simulink model "longitudinal_lateral_dynamics"  (R2024b)
settings: Solver=VariableStepAuto  StartTime=0.0  StopTime=10  RelTol=1e-3
values from neighbouring files (symbols this model uses):
  Cd = [0 1]    [mpc3.m]
  Cr = 87342    [mpc3.m]    (also in prueba_mpc.m; prueba_mpc2.m)
  Iz = 1960    [mpc3.m]    (also in prueba_mpc.m; prueba_mpc2.m)
  lf = 1.177    [mpc3.m]    (also in prueba_mpc.m; prueba_mpc2.m)
  lr = 1.358    [mpc3.m]    (also in prueba_mpc.m; prueba_mpc2.m)
  m = 1400    [mpc3.m]    (also in prueba_mpc.m; prueba_mpc2.m)
  R = 1    [prueba_mpc.m]    (also in prueba_mpc2.m)
  vx = 10    [mpc3.m]    (also in prueba_mpc.m; prueba_mpc2.m)
undefined symbols (not defined in the file or in its folder): Af, F_max, FN, g, miu, mode, mu1, mu2, mu3, steering_angle, theta
libraries: slpidlib x1
settings Model: Creator=inaki  LastModifiedBy=inaki
settings SolverCC: MaxConsecutiveMinStep=4
settings DebuggingCC: AlgebraicLoopMsg=none

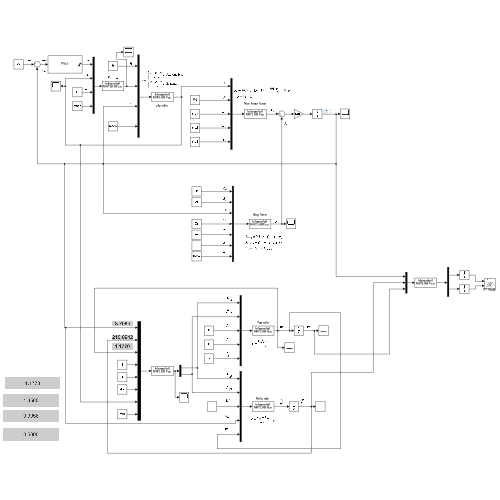
[thumbnail: Simulink's stored preview of the top-level diagram]
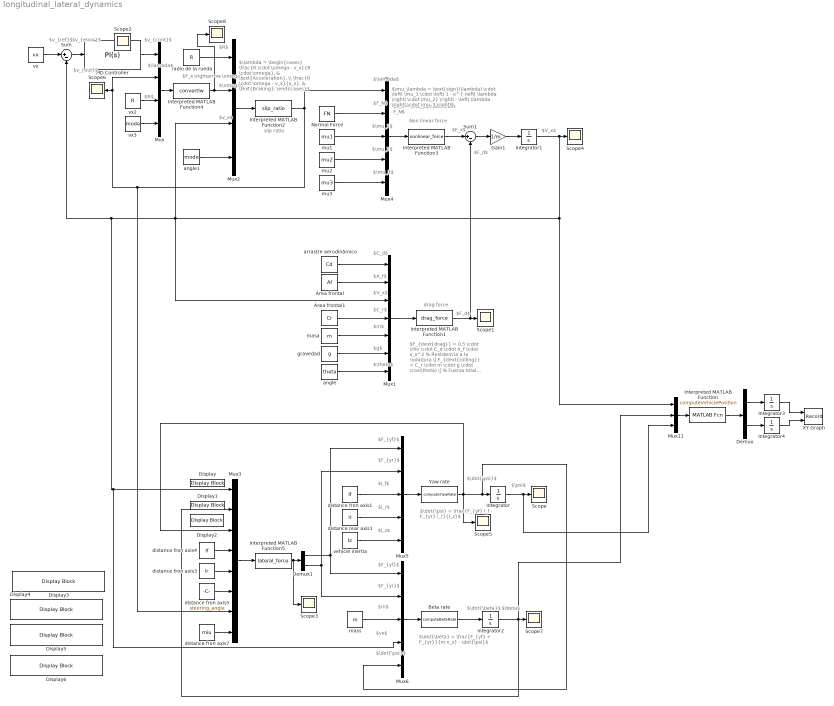
== system longitudinal_lateral_dynamics ==
  note: $v_{out}$
  note: $V_x$
  note: $V_x$
  note: $\mu_1$
  note: slip ratio
  note: $F_x \rightarrow \omega$
  note: $m$
  note: drag force
  note: $v_{error}$
  note: $C_d$
  note: $F_{\text{drag}} = 0.5 \cdot \rho \cdot C_d \cdot A_f \cdot v_x^2 % Resistencia a la rodadura \[ F_{\text{rolling}} = C_r \cdot m \cdot g \cdot \cos(\theta) \] % Fuerza total de arrastre \[ F_D = F_{\text{drag}} + F_{\text{rolling}} \]$
  note: $\lambda$
  note: $F_d$
  note: Non linear force
  note: $\omega$
  note: $F_x = \mu_\lambda \cdot F_N$
  note: $F_d$
  note: $A_f$
  note: $C_r$
  note: $v_{cont}$
  note: $g$
  note: $v_{ref}$
  note: $v_x$
  note: $\theta$
  note: $F_x$
  note: $\lambda = \begin{cases} \frac{R \cdot \omega - v_x}{R \cdot \omega}, & \text{Acceleration}, \\ \frac{R \cdot \omega - v_x}{v_x}, & \text{Braking}. \end{cases}$
  note: $R$
  note: $\lambda$
  note: $\mu_3$
  note: $\mu_\lambda = \text{sign}(\lambda) \cdot \left( \mu_1 \cdot \left( 1 - e^{-\left| \lambda \right| \cdot \mu_2} \right) - \left| \lambda \right| \cdot \mu_3 \right)$
  note: $R$
  note: $\mu_2$
  note: $F_N$
  note: $\dot{\psi}$
  note: $F_{yr}$
  note: $\dot{\beta}$
  note: $F_{yf}$
  note: $\dot{\beta} = \frac{F_{yf} + F_{yr}}{m v_x} - \dot{\psi}$
  note: $m$
  note: $\dot{\psi}$
  note: $F_{yf}$
  note: $vx$
  note: $\psi$
  note: $I_r$
  note: $\beta$
  note: $I_z$
  note: $F_{yr}$
  note: $I_f$
  note: $\dot{\psi} = \frac{F_{yf} l_f - F_{yr} l_r}{I_z}$
  Beta rate : MATLABFcn  MATLABFcn=computeBetaRate
  Demux : Demux  Outputs=2
  Demux1 : Demux  Outputs=2
  Display{,1,3..6} (6 alike) : DisplayBlock  LabelPosition=Hide  Transparency=1
  Display2 : DisplayBlock  LabelPosition=Hide  Transparency=1  Layout=Fill available space
  Gain1 : Gain  Gain=1/m
  Integrator{,1..4} (5 alike) : Integrator
  Interpreted MATLAB Function : MATLABFcn  MATLABFcn=computeVehiclePosition
  Interpreted MATLAB Function1 : MATLABFcn  MATLABFcn=drag_force  Output1D=off
  Interpreted MATLAB Function2 : MATLABFcn  MATLABFcn=slip_ratio  Output1D=off
  Interpreted MATLAB Function3 : MATLABFcn  MATLABFcn=nonlinear_force  Output1D=off
  Interpreted MATLAB Function4 : MATLABFcn  MATLABFcn=convertlw  OutputDimensions=1  Output1D=off
  Interpreted MATLAB Function5 : MATLABFcn  MATLABFcn=lateral_force  OutputDimensions=2
  Mux : Mux
  Mux1 : Mux  Inputs=7
  Mux11 : Mux  Inputs=3
  Mux2 : Mux
  Mux3 : Mux  Inputs=8
  Mux4 : Mux  Inputs=5
  Mux5 : Mux  Inputs=5
  Mux6 : Mux  Inputs=5
  Normal Force : Constant  Value=FN
  PID Controller : slpidlib/PID Controller  Controller=PI  Form=Parallel  TimeDomain=Continuous-time  UseExternalTs=off  SampleTime=-1  IntegratorMethod=Forward Euler  FilterMethod=Forward Euler  ControllerParametersSource=internal  P=3371.8  I=1668.7038  UseKiTs=off  D=0  UseExternalDerivativeSource=off  N=100  UseFilter=on  TunerSelectOption=Transfer Function Based (PID Tuner App)  InitialConditionSource=internal  InitialConditionForIntegrator=0  InitialConditionForFilter=0  DifferentiatorICPrevScaledInput=0  ExternalReset=none  TrackingMode=off  Kt=1  LimitOutput=on  SatLimitsSource=internal  UpperSaturationLimit=F_max  LowerSaturationLimit=-F_max  LinearizeAsGain=on  AntiWindupMode=clamping  Kb=1  LimitIntegrator=off  UpperIntegratorSaturationLimit=inf  LowerIntegratorSaturationLimit=-inf  POutMin=[]  POutMax=[]  IOutMin=[]  IOutMax=[]  DOutMin=[]  DOutMax=[]  NOutMin=[]  NOutMax=[]  SumOutMin=[]  SumOutMax=[]  SaturationOutMin=[]  SaturationOutMax=[]  PParamMin=[]  PParamMax=[]  IParamMin=[]  IParamMax=[]  DParamMin=[]  DParamMax=[]  NParamMin=[]  NParamMax=[]  KbParamMin=[]  KbParamMax=[]  KtParamMin=[]  KtParamMax=[]  KbOutMin=[]  KbOutMax=[]  KtOutMin=[]  KtOutMax=[]  IntegratorOutMin=[]  IntegratorOutMax=[]  FilterOutMin=[]  FilterOutMax=[]  SumI1OutMin=[]  SumI1OutMax=[]  SumI2OutMin=[]  SumI2OutMax=[]  SumI3OutMin=[]  SumI3OutMax=[]  SumI4OutMin=[]  SumI4OutMax=[]  SumDOutMin=[]  SumDOutMax=[]  DifferentiatorOutMin=[]  DifferentiatorOutMax=[]  FilterDiffOutCoefMin=[]  FilterDiffOutCoefMax=[]  ReciprocalOutMin=[]  ReciprocalOutMax=[]  SumDenOutMin=[]  SumDenOutMax=[]  SumNumOutMin=[]  SumNumOutMax=[]  DivideOutMin=[]  DivideOutMax=[]  UdiffTsProdOutMin=[]  UdiffTsProdOutMax=[]  NTsProdOutMin=[]  NTsProdOutMax=[]  UintegralTsProdOutMin=[]  UintegralTsProdOutMax=[]  UngainTsProdOutMin=[]  UngainTsProdOutMax=[]  ClampingZeroOutDataTypeStr=Inherit: Inherit via back propagation  ClampingZeroOutMin=[]  ClampingZeroOutMax=[]  FilterDenConstantOutDataTypeStr=Inherit: Inherit via back propagation  FilterDenConstantOutMin=[]  FilterDenConstantOutMax=[]  PCopyOutDataTypeStr=Inherit: Inherit via back propagation  PCopyOutMin=[]  PCopyOutMax=[]  NCopyOutDataTypeStr=Inherit: Inherit via back propagation  NCopyOutMin=[]  NCopyOutMax=[]  IntegratorContinuousStateAttributes=''  IntegratorStateMustResolveToSignalObject=off  IntegratorRTWStateStorageClass=Auto  FilterContinuousStateAttributes=''  FilterStateMustResolveToSignalObject=off  FilterRTWStateStorageClass=Auto  ParallelPVariant=InternalParameters  IdealPVariant=Disabled  IVariant=InternalParameters  DVariant=Disabled  IntegratorVariant=Continuous  SatVariant=Enabled  AWVariant=ContClampingParallel  PCopyVariant=Disabled  TRVariant=Disabled  FdbkBlocksVariant=Forward  IdealPFdbkVariant=Disabled  SatFdbkVariant=Disabled  DerivativeFilterVariant=Disabled  NVariant=Disabled  NCopyVariant=Disabled_SignalSpec  FilterICVariant=Disabled  IntegratorICVariant=InternalICs  ExternalResetVariant=Disabled  TRSumVariant=Passthrough  SumFdbkVariant=Disabled  SumVariant=Sum_PI  TsampFilterVariant=InternalTs  TsampNgainVariant=Passthrough  TsampIntegralVariant=Disabled_SignalSpec  ExternalSaturationOutDataTypeStr=Inherit: Same as second input  DerivativeSourceVariant=Disabled  PreIntVariant=InternalPreInt
  Scope{,1..8} (9 alike) : Scope
  Sum : Sum  Inputs=|+-
  Sum1 : Sum  Inputs=|+-
  XY Graph : Record  VariableName=pos  RecordToWorkspace=on  FileSettingsInternal="{\"entries\":[{\"content\":{\"excelSettings\":{\"content\":{},\"type\":\"Streamout.ExcelSettings\"}},\"type\":\"Streamout.FileSettingStorage\",\"uuid\":\"\"}],\"packageUris\":[\"http:\\/\\/schema.mathworks.com\\/mf0\\/streamout_blocks\\/R2020a\"],\"version\":\"1.0\"}"  Layout=[1 1]  SignalsInternal="{\"entries\":[{\"content\":{\"signals\":[{\"content\":{\"blockPath\":[],\"dimensions\":[1],\"domain\":\"\",\"lineColor\":\"#a2142f\",\"plots\":[ 1 ],\"port\":1,\"sid\":[\"\"],\"signalID\":1,\"signalName\":\"Integrator3\"},\"type\":\"RecordBlkView.Signal\",\"uuid\":\"\"},{\"content\":{\"blockPath\":[],\"dimensions\":[1],\"domain\":\"\",\"lineColor\":\"#139fff\",\"plots\":[ 1 ],\"port\":2,\"sid\":[\"\"],\"signalID\":2,\"signalName\":\"Integrator4\"},\"type\":\"RecordBlkView.Signal\",\"uuid\":\"\"}]},\"type\":\"RecordBlkView.InputSignals\",\"uuid\":\"\"}],\"packageUris\":[\"http:\\/\\/schema.mathworks.com\\/mf0\\/streamout_blocks\\/R2020a\"],\"version\":\"1.0\"}"  VisualizationBindings="{\"xyplotplugin\":{\"info\":[{\"series\":[{\"bindingParametersList\":[{\"parameter\":\"X-Axis\",\"signalID\":1,\"signalName\":\"Integrator3\"},{\"parameter\":\"Y-Axis\",\"signalID\":2,\"signalName\":\"Integrator4\"}],\"seriesID\":0}],\"subplotID\":1}]}}"  CompatibilityTag=XY
  Yaw rate : MATLABFcn  MATLABFcn=computeYawRate
  angle : Constant  Value=theta  VectorParams1D=off
  angle1 : Constant  Value=mode
  arrastre aerodinámico : Constant  Value=Cd  VectorParams1D=off
  distance fron axis1 : Constant  Value=lf
  distance fron axis3 : Constant  Value=lr
  distance fron axis4 : Constant  Value=lf
  distance fron axis5 : Constant  Value=steering_angle
  distance fron axis7 : Constant  Value=miu
  distance rear axis1 : Constant  Value=lr
  gravedad : Constant  Value=g  VectorParams1D=off
  masa : Constant  Value=m  VectorParams1D=off
  mass : Constant  Value=m
  mu1 : Constant  Value=mu1
  mu2 : Constant  Value=mu2
  mu3 : Constant  Value=mu3
  radio de la rueda : Constant  Value=R  VectorParams1D=off
  vehicle inertia : Constant  Value=Iz
  vx : Constant  Value=vx  VectorParams1D=off
  vx2 : Constant  Value=R  VectorParams1D=off  SampleTime=R
  vx3 : Constant  Value=mode  VectorParams1D=off  SampleTime=mode
  Área frontal : Constant  Value=Af  VectorParams1D=off
  Área frontal1 : Constant  Value=Cr  VectorParams1D=off
  wires:
  masa/1 -> Mux1/5
  Sum1/1 -> Gain1/1
  arrastre aerodinámico/1 -> Mux1/1
  Gain1/1 -> Integrator1/1
  Sum/1 -> PID Controller/1
  Mux4/1 -> Interpreted MATLAB Function3/1
  gravedad/1 -> Mux1/6
  angle1/1 -> Mux2/4
  Interpreted MATLAB Function3/1 -> Sum1/1
  mu3/1 -> Mux4/5
  mu2/1 -> Mux4/4
  angle/1 -> Mux1/7
  Interpreted MATLAB Function1/1 -> Sum1/2, Scope1/1
  vx/1 -> Sum/1
  Mux/1 -> Interpreted MATLAB Function4/1
  PID Controller/1 -> Mux/1
  Mux2/1 -> Interpreted MATLAB Function2/1
  Interpreted MATLAB Function4/1 -> Scope8/1, Mux2/2
  radio de la rueda/1 -> Mux2/1
  Normal Force/1 -> Mux4/2
  Mux1/1 -> Interpreted MATLAB Function1/1
  Área frontal/1 -> Mux1/2
  Área frontal1/1 -> Mux1/4
  vx2/1 -> Mux/3
  vx3/1 -> Mux/4
  mu1/1 -> Mux4/3
  Mux11/1 -> Interpreted MATLAB Function/1
  Interpreted MATLAB Function/1 -> Demux/1
  Demux/1 -> Integrator3/1
  Integrator3/1 -> XY Graph/1
  Demux/2 -> Integrator4/1
  Integrator4/1 -> XY Graph/2
  distance fron axis4/1 -> Mux3/4
  vehicle inertia/1 -> Mux5/5
  distance rear axis1/1 -> Mux5/4
  distance fron axis1/1 -> Mux5/3
  distance fron axis3/1 -> Mux3/5
  distance fron axis7/1 -> Mux3/8
  Integrator2/1 -> Mux3/2, Mux11/2, Scope7/1
  Demux1/2 -> Mux5/2, Mux6/2
  Mux5/1 -> Yaw rate/1
  Interpreted MATLAB Function5/1 -> Scope3/1, Demux1/1
  Mux6/1 -> Beta rate/1
  Yaw rate/1 -> Scope5/1, Mux3/3, Mux6/5, Integrator/1
  distance fron axis5/1 -> Mux3/6
  Mux3/1 -> Interpreted MATLAB Function5/1
  Demux1/1 -> Mux5/1, Mux6/1
  mass/1 -> Mux6/3
  Beta rate/1 -> Integrator2/1
  Integrator/1 -> Mux11/3, Scope/1
  Integrator1/1 -> Mux1/3, Mux3/1, Mux6/4, Sum/2, Mux2/3, Mux11/1, Scope4/1
  Interpreted MATLAB Function2/1 -> Mux4/1, Mux/2, Scope6/1, Mux3/7
